simulink model "simulacion_lab5_2"  (R2020a)
settings: Solver=VariableStepAuto  StartTime=0.0  StopTime=10.0  RelTol=1e-3
settings Model: Creator=Miguel Gutierrez  LastModifiedBy=Miguel Gutierrez

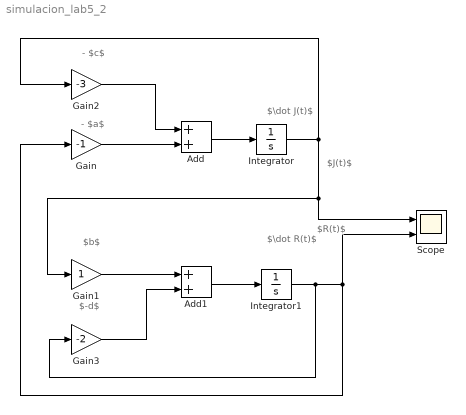
== system simulacion_lab5_2 ==
  note: $b$
  note: - $a$
  note: $\dot J(t)$
  note: $R(t)$
  note: $J(t)$
  note: $\dot R(t)$
  note: - $c$
  note: $-d$
  Add : Sum
  Add1 : Sum
  Gain : Gain  Gain=-1
  Gain1 : Gain
  Gain2 : Gain  Gain=-3
  Gain3 : Gain  Gain=-2
  Integrator : Integrator  InitialCondition=5
  Integrator1 : Integrator
  Scope : Scope  NumInputPorts=2
  wires:
  Gain/1 -> Add/2
  Gain2/1 -> Add/1
  Add/1 -> Integrator/1
  Integrator1/1 -> Gain3/1, Scope/2, Gain/1
  Gain3/1 -> Add1/2
  Gain1/1 -> Add1/1
  Add1/1 -> Integrator1/1
  Integrator/1 -> Gain1/1, Scope/1, Gain2/1
